simulink model "Question_6_Step"  (R2021a)
settings: Solver=VariableStepAuto  StartTime=0.0  StopTime=10.0  RelTol=1e-3
settings Model: Creator=haden  LastModifiedBy=haden

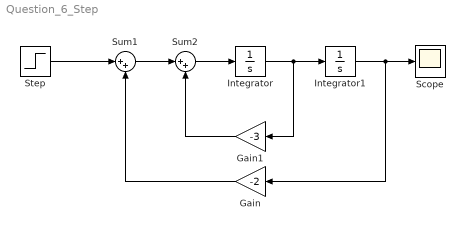
== system Question_6_Step ==
  Gain : Gain  Gain=-2
  Gain1 : Gain  Gain=-3
  Integrator : Integrator
  Integrator1 : Integrator
  Scope : Scope
  Step : Step  SampleTime=0
  Sum1 : Sum  Inputs=|++
  Sum2 : Sum  Inputs=|++
  wires:
  Integrator/1 -> Gain1/1, Integrator1/1
  Gain/1 -> Sum1/2
  Integrator1/1 -> Scope/1, Gain/1
  Gain1/1 -> Sum2/2
  Sum2/1 -> Integrator/1
  Sum1/1 -> Sum2/1
  Step/1 -> Sum1/1
